simulink model "SeriesExcited_model"  (R2024a)
settings: Solver=VariableStepAuto  StartTime=0.0  StopTime=50  RelTol=1e-3
undefined symbols (not defined in the file or in its folder): B1, dt, dT, J1, La1, Lf1, LoadMode, Ra1, Rf1, Ro, SlopeR, Ts, Vp, Vs
libraries: simulink x1
settings Model: Creator=Xuan  LastModifiedBy=admin
settings RTWCC: GPUComputeCapability=3.5

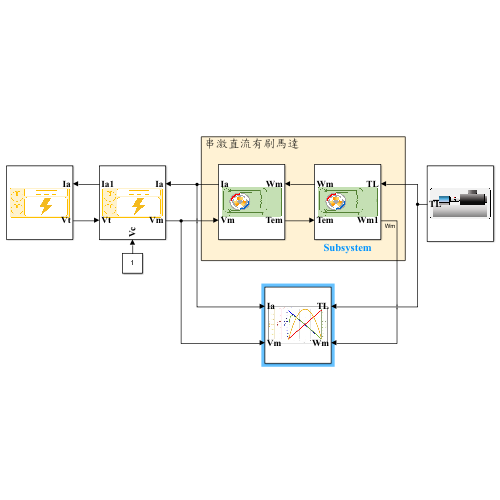
[thumbnail: Simulink's stored preview of the top-level diagram]
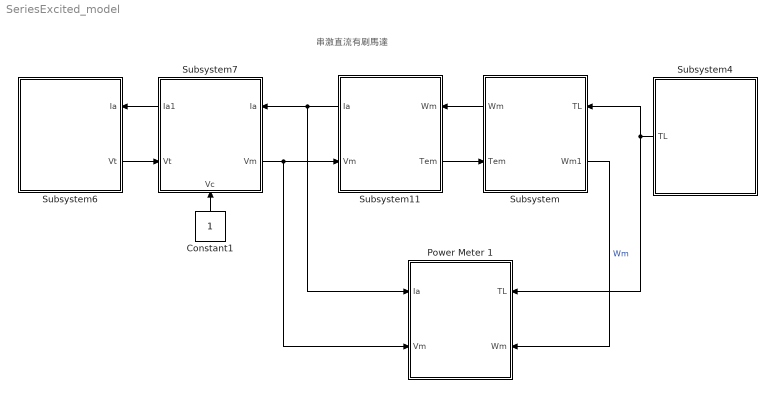
== system SeriesExcited_model ==
  note: 串激直流有刷馬達
  Constant1 : Constant
  Power Meter 1 : Subsystem  InitFcn=|  StopFcn=|
      InitFcn=|
      | %% ModePlot
      | % PlotMode=1 or 2
      | PlotMode = 2;
      StopFcn=|
      | % %% Data Loading
      | % 
      | % tl1 = out.Tl1;
      | % f1 = size(tl1);
      | % 
      | % % clear datas 
      | % torque1 = 0;
      | % x11 = 0;
      | % y11 = 0; y21 = 0; y31 = 0; y41 = 0; y51 = 0; y61 = 0;
      | % 
      | % switch LoadMode   % mode ( 1:ramp load , 2:stair load )
      | % 
      | %     case 1  
      | % 
      | %         i = 1;
      | %         while 1
      | %             if tl1(i) > 0.01
      | %                s = i;
      | %                break
      | %             end
      | %             i = i+1;
      | %         end
      | %         torque1 = out.Tl1(s:f1(1));
      | %         x11 = out.omega1(s:f1(1));
      | %         % y11 = out.omega1(s:f1(1));
      | %         y21 = out.Eff1(s:f1(1));
      | %         y31 = out.Pin1(s:f1(1));
      | %         y41 = out.Pout1(s:f1(1));
      | %         y51 = out.Vs(s:f1(1));
      | %         y61 = out.Ia1(s:f1(1));
      | %         case 2
      | % 
      | %         tl_pre1 = 0;
      | %         j = 1;
      | %         for i = 1:f1(1)           
      | %             if tl1(i) > tl_pre1
      | %                 torque1(j,1) = tl1(i-1);
      | %                 x11(j,1) = out.omega1((i-1),1);
      | %                 % y11(j,1) = out.omega1((i-1),1);
      | %                 y21(j,1) = out.Eff1((i-1),1);
      | %                 y31(j,1) = out.Pin1((i-1),1);
      | %                 y41(j,1) = out.Pout1((i-1),1);
      | %                 y51(j,1) = out.Vs((i-1),1);
      | %                 y61(j,1) = out.Ia1((i-1),1);
      | %                 j = j+1;
      | %             end
      | %             tl_pre1 = tl1(i);
      | %         end
      | % end
      | % 
      | % %% Plot
      | % % plot TN curve
      | % 
      | % % figure(1);
      | % 
      | % figure(2);
      | % set(gcf, 'Position', [1050, 300, 1000, 500]); % [left, bottom, width, height]
      | % clf;
      | % 
      | % % Create empty axis system with 4 y axis by calling:
      | % % handle = maxis(number of axis, y-spacing between outside lines)
      | % h = myaxisc(5,0.10,[0.1,0.1,0.8,0.8]); % Specify position
      | % 
      | % % Call plot and specify y-axis number using method h.p(nr). For creating a
      | % % legend later, we need to assign the handles returned by plot to p.
      | % switch PlotMode
      | % 
      | %     case 1  
      | %         p(1) = plot(h.p(1),x11,torque1,'b','LineWidth',1.2);
      | %         p(2) = plot(h.p(2),x11,y21,'Color',[0.4660 0.6740 0.1880],'LineWidth',1.2);
      | %         p(3) = plot(h.p(3),x11,y61,'Color',[0.3010 0.7450 0.9330],'LineWidth',1.2);
      | %         p(4) = plot(h.p(4),x11,y51,'r','LineWidth',1.2);
      | %         p(5) = plot(h.p(5),x11,y31,'m','LineWidth',1.2);
      | %         print("case1");
      | % 
      | %     case 2
      | %         p(1) = plot(h.p(1),x11,torque1,'b-*','LineWidth',1.1);
      | %         p(2) = plot(h.p(2),x11,y21,'-*','Color',[0.4660 0.6740 0.1880],'LineWidth',1.1);
      | %         p(3) = plot(h.p(3),x11,y61,'-*','Color',[0.3010 0.7450 0.9330],'LineWidth',1.1);
      | %         p(4) = plot(h.p(4),x11,y51,'r-*','LineWidth',1.1);
      | %         p(5) = plot(h.p(5),x11,y31,'m-*','LineWidth',1.1);
      | %         print("case2");
      | % 
      | % end
      | % 
      | % h.autoscale % Automatically Scale Y Axis
      | % 
      | % % Additional methods to modify appearance, scaling and so on:
      | % 
      | % h.autoy(3) % Autoscale only specified y-axis
      | % %h.ylim(3,[95,105]); % Set Y-Limits for axis 3
      | % l = size(torque1);
      | % h.xlim([min(x11),max(x11)+50]);
      | % h.ylim(2,[0,100]); % Set Y-Limits for axis 4
      | % 
      | % h.gridon % Enable grid (use h.gridoff to remove)
      | % 
      | % % Modify the y-Axis Color
      | % h.ycolor(1,'b'); % torque
      | % h.ycolor(2,[0.4660 0.6740 0.1880]); % efficiency
      | % h.ycolor(3,[0.3010 0.7450 0.9330]); % current
      | % h.ycolor(4,'r'); % voltage
      | % h.ycolor(5,'m'); % power in
      | % 
      | % % Add y-Labels
      | % % h.ylabel(1,'Speed (RPM)');
      | % h.ylabel(1, 'TL (Nm)');
      | % h.ylabel(2,'Efficiency (%)');
      | % h.ylabel(3,'Current (A)');
      | % h.ylabel(4,'Voltage (volt)');
      | % h.ylabel(5,'Pin (W)');
      | % 
      | % % Add x-Label
      | % % h.xlabel('TL (Nm)');
      | % h.xlabel('Speed (RPM)');
      | % 
      | % % Add title
      | % title('TNcurve of Series Excited Motor');
      | % set(gca,'FontWeight','bold','FontSize',14);
      | % 
      | % % Change Position of the whole myaxisc-Object
      | % h.position([0.1,0.1,0.8,0.8],0.12); % Position-Vector and Spacing 0.12
      | % 
      | % % Change all font sizes
      | % h.fontsize(10)
      | % 
      | % %% DataSaving
      | % time = out.tout;
      | % powerin1 = out.Pin1;
      | % powerout1 = out.Pout1;
      | % speed1 = out.omega1;
      | % efficiency1 = out.Eff1;
      | % voltage1 = out.Vs;
      | % current1 = out.Ia1;
      | % 
      | % filename = 'Series_TNcurve_DataSave.csv';
      | % savedata = [time, powerin1, powerout1, speed1, efficiency1, voltage1, current1];
      | % writematrix(savedata, filename);
      settings: PortSchema="{\"entries\":[{\"content\":{\"sides\":[{\"content\":{\"connectorIds\":[\"In1\",\"In2\"]},\"type\":\"ConnectorPlacement.EquallySpacedRectSide\",\"uuid\":\"e8c36156-32d4-4676-af0d-0891e0773ccb\"},{\"content\":{\"connectorIds\":[\"In3\",\"In4\"],\"side\":\"RIGHT\"},\"type\":\"ConnectorPlacement.EquallySpacedRectSide\",\"uuid\":\"5c876be3-b715-4990-b5f5-1fbda74411c9\"},{\"content\":{\"side\":\"TOP\"},\"type\":\"ConnectorPlacement.EquallySpacedRectSide\",\"uuid\":\"8aaa78a6-3767-49bf-860f-056d8a2101ef\"}]},\"type\":\"ConnectorPlacement.EquallySpacedConnector\",\"uuid\":\"6a38af7a-9eb4-49af-a88b-27cf70b05ead\"}],\"packageUris\":[\"http://schema.mathworks.com/mf0/Connector/R2020b\"],\"version\":\"1.0\"}"
      mask Display: image('TNcurve2.png');
  Subsystem : Subsystem  InitFcn=|
      | J1 = 0.008;
      | B1 = 0.0015;
      settings: PortSchema="{\"entries\":[{\"content\":{\"sides\":[{\"content\":{\"connectorIds\":[\"Out2\",\"In1\"]},\"type\":\"ConnectorPlacement.EquallySpacedRectSide\",\"uuid\":\"f01d68ef-b57c-407d-be4c-54b43c4822fb\"},{\"content\":{\"connectorIds\":[\"In2\",\"Out1\"],\"side\":\"RIGHT\"},\"type\":\"ConnectorPlacement.EquallySpacedRectSide\",\"uuid\":\"a6b4f32d-c627-4c5c-aa56-157e24ac13be\"},{\"content\":{\"side\":\"TOP\"},\"type\":\"ConnectorPlacement.EquallySpacedRectSide\",\"uuid\":\"54a4d4d6-c45c-4cfb-8847-3e2e340fdc5a\"}]},\"type\":\"ConnectorPlacement.EquallySpacedConnector\",\"uuid\":\"c9ccd625-7413-4435-9b22-3277d2f45bfd\"}],\"packageUris\":[\"http://schema.mathworks.com/mf0/Connector/R2020b\"],\"version\":\"1.0\"}"
      mask Display: image('直流串激馬達2.png');
  Subsystem11 : Subsystem  InitFcn=|
      | La1 = 0.0082;
      | Ra1 = 0.035;
      | Lf1 = 0.0014;
      | Rf1 = 0.165;
      settings: PortSchema="{\"entries\":[{\"content\":{\"sides\":[{\"content\":{\"connectorIds\":[\"Out2\",\"In1\"]},\"type\":\"ConnectorPlacement.EquallySpacedRectSide\",\"uuid\":\"f01d68ef-b57c-407d-be4c-54b43c4822fb\"},{\"content\":{\"connectorIds\":[\"In2\",\"Out1\"],\"side\":\"RIGHT\"},\"type\":\"ConnectorPlacement.EquallySpacedRectSide\",\"uuid\":\"a6b4f32d-c627-4c5c-aa56-157e24ac13be\"},{\"content\":{\"side\":\"TOP\"},\"type\":\"ConnectorPlacement.EquallySpacedRectSide\",\"uuid\":\"54a4d4d6-c45c-4cfb-8847-3e2e340fdc5a\"}]},\"type\":\"ConnectorPlacement.EquallySpacedConnector\",\"uuid\":\"c9ccd625-7413-4435-9b22-3277d2f45bfd\"}],\"packageUris\":[\"http://schema.mathworks.com/mf0/Connector/R2020b\"],\"version\":\"1.0\"}"
      mask Display: image('直流串激馬達2.png');
  Subsystem4 : Subsystem  InitFcn=|
      | dt = 0.2;
      | dT = 0.05;
      | Ts = 2;
      | SlopeR = 0.2;
      | % if LoadMode>1.5, then use stair load
      | % if LoadMode<1.5, use linear load
      | LoadMode = 2;
      mask Display: image('主動式動力機2.png');
  Subsystem6 : Subsystem  InitFcn=|
      | Vs = 48;
      | Ro = 0.001;
      settings: PortSchema="{\"entries\":[{\"content\":{\"sides\":[{\"content\":{},\"type\":\"ConnectorPlacement.EquallySpacedRectSide\",\"uuid\":\"717e91a0-288b-4ba5-84da-f262c24688bc\"},{\"content\":{\"connectorIds\":[\"In1\",\"Out1\"],\"side\":\"RIGHT\"},\"type\":\"ConnectorPlacement.EquallySpacedRectSide\",\"uuid\":\"569ee505-38fb-400b-9e45-0fafedafb0f3\"},{\"content\":{\"side\":\"TOP\"},\"type\":\"ConnectorPlacement.EquallySpacedRectSide\",\"uuid\":\"44407c3d-239d-4fc9-b2d2-10ddbad2f525\"}]},\"type\":\"ConnectorPlacement.EquallySpacedConnector\",\"uuid\":\"e894aa65-7991-48d5-91da-50bab94327d3\"}],\"packageUris\":[\"http://schema.mathworks.com/mf0/Connector/R2020b\"],\"version\":\"1.0\"}"
      mask Display: image('直流電源2.png', "center");
  Subsystem7 : Subsystem  InitFcn=Vp = 1;
      settings: PortSchema="{\"entries\":[{\"content\":{\"sides\":[{\"content\":{\"connectorIds\":[\"Out2\",\"In1\"]},\"type\":\"ConnectorPlacement.EquallySpacedRectSide\",\"uuid\":\"717e91a0-288b-4ba5-84da-f262c24688bc\"},{\"content\":{\"connectorIds\":[\"In3\",\"Out1\"],\"side\":\"RIGHT\"},\"type\":\"ConnectorPlacement.EquallySpacedRectSide\",\"uuid\":\"569ee505-38fb-400b-9e45-0fafedafb0f3\"},{\"content\":{\"side\":\"TOP\"},\"type\":\"ConnectorPlacement.EquallySpacedRectSide\",\"uuid\":\"44407c3d-239d-4fc9-b2d2-10ddbad2f525\"},{\"content\":{\"connectorIds\":[\"In2\"],\"side\":\"BOTTOM\"},\"type\":\"ConnectorPlacement.EquallySpacedRectSide\",\"uuid\":\"abc944a0-1837-407a-a5f0-1c34ab870232\"}]},\"type\":\"ConnectorPlacement.EquallySpacedConnector\",\"uuid\":\"e894aa65-7991-48d5-91da-50bab94327d3\"}],\"packageUris\":[\"http://schema.mathworks.com/mf0/Connector/R2020b\"],\"version\":\"1.0\"}"
      mask Display: image('直流電源2.png');
  wires:
  Subsystem11/1(Tem) -> Subsystem/1(Tem)
  Subsystem/2(Wm) -> Subsystem11/2(Wm)
  Subsystem7/2(Ia1) -> Subsystem6/1(Ia)
  Subsystem6/1(Vt) -> Subsystem7/1(Vt)
  Subsystem11/2(Ia) -> Power Meter 1/1(Ia), Subsystem7/3(Ia)
  Subsystem7/1(Vm) -> Power Meter 1/2(Vm), Subsystem11/1(Vm)
  Subsystem4/1(TL) -> Power Meter 1/3(TL), Subsystem/2(TL)
  Subsystem/1(Wm1) -> Power Meter 1/4(Wm)  "Wm"
  Constant1/1 -> Subsystem7/2(Vc)

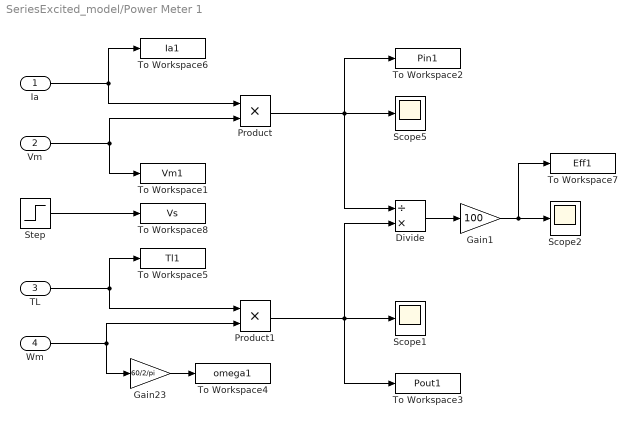
== system SeriesExcited_model/Power Meter 1 ==
  Ia : Inport
  Vm : Inport  Port=2
  TL : Inport  Port=3
  Wm : Inport  Port=4
  Divide : Product  Inputs=/*
  Gain1 : Gain  Gain=100
  Gain23 : Gain  Gain=60/2/pi
  Product : Product
  Product1 : Product
  Scope1 : Scope
  Scope2 : Scope
  Scope5 : Scope
  Step : Step  Time=0.1  After=Vs  SampleTime=0
  To Workspace1 : ToWorkspace  VariableName=Vm1  SampleTime=-1
  To Workspace2 : ToWorkspace  VariableName=Pin1  SampleTime=-1
  To Workspace3 : ToWorkspace  VariableName=Pout1  SampleTime=-1
  To Workspace4 : ToWorkspace  VariableName=omega1  SampleTime=-1
  To Workspace5 : ToWorkspace  VariableName=Tl1  SampleTime=-1
  To Workspace6 : ToWorkspace  VariableName=Ia1  SampleTime=-1
  To Workspace7 : ToWorkspace  VariableName=Eff1  SampleTime=-1
  To Workspace8 : ToWorkspace  VariableName=Vs  SampleTime=-1
  wires:
  Gain1/1 -> Scope2/1, To Workspace7/1
  Divide/1 -> Gain1/1
  Gain23/1 -> To Workspace4/1
  Wm/1 -> Gain23/1, Product1/2
  TL/1 -> Product1/1, To Workspace5/1
  Product1/1 -> Divide/2, To Workspace3/1, Scope1/1
  Product/1 -> To Workspace2/1, Scope5/1, Divide/1
  Vm/1 -> Product/2, To Workspace1/1
  Ia/1 -> To Workspace6/1, Product/1
  Step/1 -> To Workspace8/1

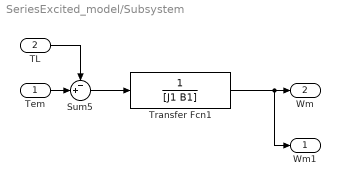
== system SeriesExcited_model/Subsystem ==
  Tem : Inport
  TL : Inport  Port=2
  Sum5 : Sum  Inputs=-+|
  Transfer Fcn1 : TransferFcn  Denominator=[J1 B1]
  Wm1 : Outport
  Wm : Outport  Port=2
  wires:
  Transfer Fcn1/1 -> Wm/1, Wm1/1
  Tem/1 -> Sum5/2
  TL/1 -> Sum5/1
  Sum5/1 -> Transfer Fcn1/1

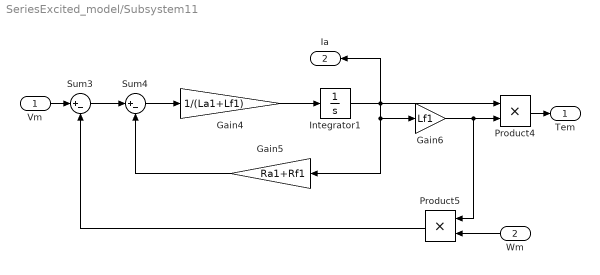
== system SeriesExcited_model/Subsystem11 ==
  Vm : Inport
  Wm : Inport  Port=2
  Gain4 : Gain  Gain=1/(La1+Lf1)
  Gain5 : Gain  Gain=Ra1+Rf1
  Gain6 : Gain  Gain=Lf1
  Integrator1 : Integrator
  Product4 : Product
  Product5 : Product
  Sum3 : Sum  Inputs=|+-
  Sum4 : Sum  Inputs=|+-
  Tem : Outport
  Ia : Outport  Port=2
  wires:
  Product4/1 -> Tem/1
  Vm/1 -> Sum3/1
  Gain5/1 -> Sum4/2
  Sum3/1 -> Sum4/1
  Product5/1 -> Sum3/2
  Sum4/1 -> Gain4/1
  Gain6/1 -> Product5/1, Product4/2
  Gain4/1 -> Integrator1/1
  Integrator1/1 -> Gain5/1, Gain6/1, Product4/1, Ia/1
  Wm/1 -> Product5/2

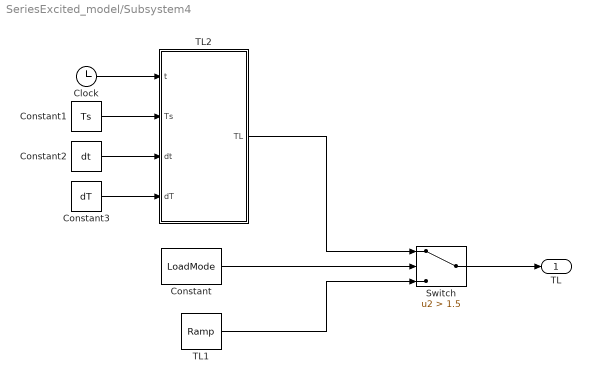
== system SeriesExcited_model/Subsystem4 ==
  Clock : Clock
  Constant : Constant  Value=LoadMode
  Constant1 : Constant  Value=Ts
  Constant2 : Constant  Value=dt  SampleTime=dT
  Constant3 : Constant  Value=dT
  Switch : Switch  Criteria=u2 > Threshold  Threshold=1.5  SaturateOnIntegerOverflow=off  InputSameDT=off
  TL1 : simulink/Sources/Ramp  slope=SlopeR  start=Ts  InitialOutput=0
  TL2 : MATLAB Function  TreatAsAtomicUnit=on
  TL : Outport
  wires:
  TL1/1 -> Switch/3
  TL2/1(TL) -> Switch/1
  Constant/1 -> Switch/2
  Switch/1 -> TL/1
  Constant1/1 -> TL2/2(Ts)
  Clock/1 -> TL2/1(t)
  Constant3/1 -> TL2/4(dT)
  Constant2/1 -> TL2/3(dt)

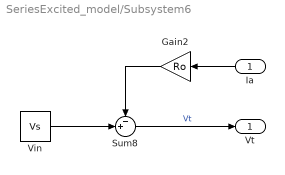
== system SeriesExcited_model/Subsystem6 ==
  Ia : Inport
  Gain2 : Gain  Gain=Ro
  Sum8 : Sum  Inputs=-+|
  Vin : Constant  Value=Vs
  Vt : Outport
  wires:
  Ia/1 -> Gain2/1
  Vin/1 -> Sum8/2
  Sum8/1 -> Vt/1  "Vt"
  Gain2/1 -> Sum8/1

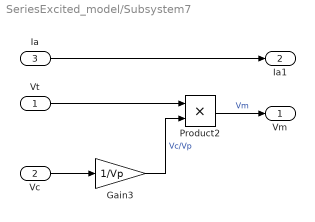
== system SeriesExcited_model/Subsystem7 ==
  Vt : Inport
  Vc : Inport  Port=2
  Ia : Inport  Port=3
  Gain3 : Gain  Gain=1/Vp
  Product2 : Product
  Vm : Outport
  Ia1 : Outport  Port=2
  wires:
  Gain3/1 -> Product2/2  "Vc/Vp"
  Product2/1 -> Vm/1  "Vm"
  Vt/1 -> Product2/1
  Vc/1 -> Gain3/1
  Ia/1 -> Ia1/1

== matlab function SeriesExcited_model/Subsystem4/TL2 ==
  data: t input; Ts input; TL output; dt input; dT input
function TL = fcn(t, Ts, dt, dT)

if t >= Ts
        TL = dT * fix((t-Ts)/dt);
else
    TL = 0;
end
